simulink model "SingleTrack"  (Simulink 8.7)
settings: Solver=ode45  SolverMode=SingleTasking  StartTime=0.0  StopTime=inf  FixedStep=0.001  RelTol=1e-3
PreLoadFcn:
  | SingleTrack_params
undefined symbols (not defined in the file or in its folder): Car_Bdy1_mass, Car_Steering_i, Car_Whl_Radius, Car_WhlBaseF, Car_WhlBaseR, mEngineMax, PT_DL_iDiff, PT_GearBox_iForwardGears
libraries: CarMaker4SL x5
(part 2 of 4)

== system SingleTrack/CarMaker/Vehicle/IPG Vehicle/Brake/CreateBus Vhcl.Wheel.PT ==
  In : Inport
  BusCreator1 : BusCreator  Inputs=20
  Demux1 : Demux  Outputs=20
  Out : Outport
  wires:
  Demux1/20 -> BusCreator1/20  "Vhcl Trq_DriveSrc_trg d3"
  Demux1/19 -> BusCreator1/19  "Vhcl Trq_DriveSrc_trg d2"
  Demux1/18 -> BusCreator1/18  "Vhcl Trq_DriveSrc_trg d1"
  Demux1/17 -> BusCreator1/17  "Vhcl Trq_DriveSrc_trg d0"
  Demux1/16 -> BusCreator1/16  "Vhcl Wheel RR WhlBearing"
  Demux1/15 -> BusCreator1/15  "Vhcl Wheel RR Trq_T2W"
  Demux1/14 -> BusCreator1/14  "Vhcl Wheel RR Trq_BrakeReg_trg"
  Demux1/13 -> BusCreator1/13  "Vhcl Wheel RR Trq_Brake"
  Demux1/12 -> BusCreator1/12  "Vhcl Wheel RL WhlBearing"
  Demux1/11 -> BusCreator1/11  "Vhcl Wheel RL Trq_T2W"
  Demux1/10 -> BusCreator1/10  "Vhcl Wheel RL Trq_BrakeReg_trg"
  Demux1/9 -> BusCreator1/9  "Vhcl Wheel RL Trq_Brake"
  Demux1/8 -> BusCreator1/8  "Vhcl Wheel FR WhlBearing"
  Demux1/7 -> BusCreator1/7  "Vhcl Wheel FR Trq_T2W"
  Demux1/6 -> BusCreator1/6  "Vhcl Wheel FR Trq_BrakeReg_trg"
  Demux1/5 -> BusCreator1/5  "Vhcl Wheel FR Trq_Brake"
  Demux1/4 -> BusCreator1/4  "Vhcl Wheel FL WhlBearing"
  Demux1/3 -> BusCreator1/3  "Vhcl Wheel FL Trq_T2W"
  Demux1/2 -> BusCreator1/2  "Vhcl Wheel FL Trq_BrakeReg_trg"
  Demux1/1 -> BusCreator1/1  "Vhcl Wheel FL Trq_Brake"
  BusCreator1/1 -> Out/1
  In/1 -> Demux1/1

== system SingleTrack/CarMaker/Vehicle/IPG Vehicle/CarAndTrailer/CarAndTrailerUpd ==
  Sync_In : Inport
  Vhcl.Steering : Inport  Port=2
  Vhcl.Motion : Inport  Port=3
  Vhcl.PoI : Inport  Port=4
  Vhcl.Wheel.FL : Inport  Port=5
  Vhcl.Wheel.FR : Inport  Port=6
  Vhcl.Wheel.RL : Inport  Port=7
  Vhcl.Wheel.RR : Inport  Port=8
  Car.Hitch.FrcTrq : Inport  Port=9
  Vhcl.Fr1A : Inport  Port=10
  CarAndTrailerUpd : S-Function  FunctionName=CM_Sfun  Parameters='CarAndTrUpd'  SFunctionDeploymentMode=off  EnableBusSupport=off
  CreateBus Brake.IF.In : Subsystem
  Sync_Out : Outport
  Brake.IF.In : Outport  Port=2
  wires:
  Vhcl.Fr1A/1 -> CarAndTrailerUpd/10  "user vehicle only"
  Vhcl.Steering/1 -> CarAndTrailerUpd/2
  Vhcl.Motion/1 -> CarAndTrailerUpd/3
  Vhcl.PoI/1 -> CarAndTrailerUpd/4
  Vhcl.Wheel.FL/1 -> CarAndTrailerUpd/5
  Vhcl.Wheel.FR/1 -> CarAndTrailerUpd/6
  Car.Hitch.FrcTrq/1 -> CarAndTrailerUpd/9
  Vhcl.Wheel.RR/1 -> CarAndTrailerUpd/8
  Vhcl.Wheel.RL/1 -> CarAndTrailerUpd/7
  CarAndTrailerUpd/2 -> CreateBus Brake.IF.In/1(In)
  CreateBus Brake.IF.In/1(Out) -> Brake.IF.In/1
  CarAndTrailerUpd/1 -> Sync_Out/1
  Sync_In/1 -> CarAndTrailerUpd/1

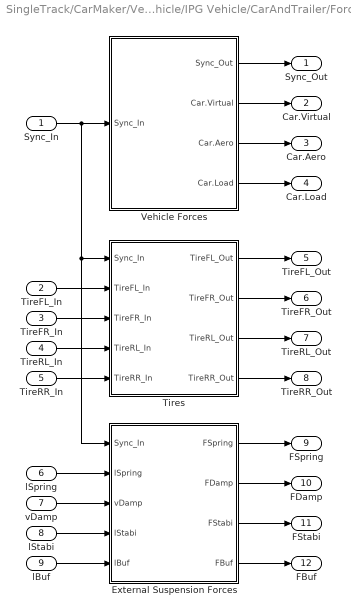
== system SingleTrack/CarMaker/Vehicle/IPG Vehicle/CarAndTrailer/Forces ==
  Sync_In : Inport
  TireFL_In : Inport  Port=2
  TireFR_In : Inport  Port=3
  TireRL_In : Inport  Port=4
  TireRR_In : Inport  Port=5
  lSpring : Inport  Port=6
  vDamp : Inport  Port=7
  lStabi : Inport  Port=8
  lBuf : Inport  Port=9
  External Suspension Forces : Subsystem
  Tires : Subsystem
  Vehicle Forces : Subsystem
  Sync_Out : Outport
  Car.Virtual : Outport  Port=2
  Car.Aero : Outport  Port=3
  Car.Load : Outport  Port=4
  TireFL_Out : Outport  Port=5
  TireFR_Out : Outport  Port=6
  TireRL_Out : Outport  Port=7
  TireRR_Out : Outport  Port=8
  FSpring : Outport  Port=9
  FDamp : Outport  Port=10
  FStabi : Outport  Port=11
  FBuf : Outport  Port=12
  wires:
  lBuf/1 -> External Suspension Forces/5(lBuf)
  lStabi/1 -> External Suspension Forces/4(lStabi)
  vDamp/1 -> External Suspension Forces/3(vDamp)
  Tires/4(TireRR_Out) -> TireRR_Out/1
  Tires/3(TireRL_Out) -> TireRL_Out/1
  Tires/2(TireFR_Out) -> TireFR_Out/1
  Tires/1(TireFL_Out) -> TireFL_Out/1
  TireRR_In/1 -> Tires/5(TireRR_In)
  TireRL_In/1 -> Tires/4(TireRL_In)
  TireFR_In/1 -> Tires/3(TireFR_In)
  TireFL_In/1 -> Tires/2(TireFL_In)
  External Suspension Forces/4(FBuf) -> FBuf/1
  Sync_In/1 -> External Suspension Forces/1(Sync_In), Tires/1(Sync_In), Vehicle Forces/1(Sync_In)
  Vehicle Forces/1(Sync_Out) -> Sync_Out/1
  Vehicle Forces/2(Car.Virtual) -> Car.Virtual/1
  Vehicle Forces/3(Car.Aero) -> Car.Aero/1
  Vehicle Forces/4(Car.Load) -> Car.Load/1
  lSpring/1 -> External Suspension Forces/2(lSpring)
  External Suspension Forces/2(FDamp) -> FDamp/1
  External Suspension Forces/3(FStabi) -> FStabi/1
  External Suspension Forces/1(FSpring) -> FSpring/1

== system SingleTrack/CarMaker/Vehicle/IPG Vehicle/CarAndTrailer/Kinematics ==
  Sync_In : Inport
  Steer.IF : Inport  Port=2
  Kinematics : S-Function  FunctionName=CM_Sfun  Parameters='Kinematics'  SFunctionDeploymentMode=off  EnableBusSupport=off
  Sync_Out : Outport
  TireFL_In : Outport  Port=2
  TireFR_In : Outport  Port=3
  TireRL_In : Outport  Port=4
  TireRR_In : Outport  Port=5
  lSpring : Outport  Port=6
  vDamp : Outport  Port=7
  lStabi : Outport  Port=8
  lBuf : Outport  Port=9
  wires:
  Kinematics/9 -> lBuf/1
  Kinematics/8 -> lStabi/1
  Kinematics/2 -> TireFL_In/1
  Kinematics/3 -> TireFR_In/1
  Kinematics/4 -> TireRL_In/1
  Kinematics/5 -> TireRR_In/1
  Kinematics/6 -> lSpring/1
  Kinematics/7 -> vDamp/1
  Sync_In/1 -> Kinematics/1
  Kinematics/1 -> Sync_Out/1
  Steer.IF/1 -> Kinematics/2

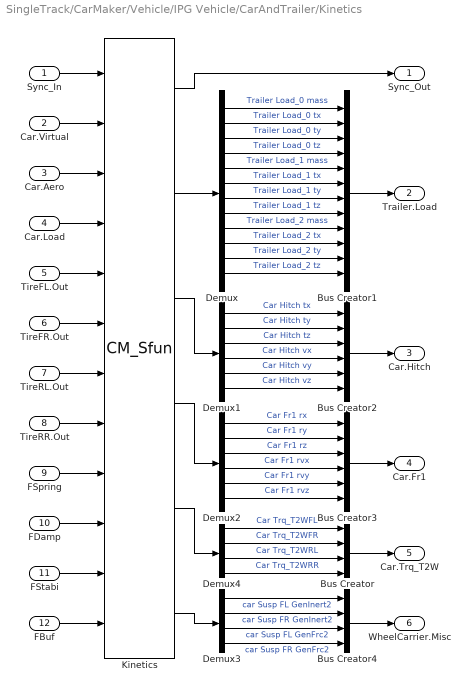
== system SingleTrack/CarMaker/Vehicle/IPG Vehicle/CarAndTrailer/Kinetics ==
  Sync_In : Inport
  Car.Virtual : Inport  Port=2
  Car.Aero : Inport  Port=3
  Car.Load : Inport  Port=4
  TireFL.Out : Inport  Port=5
  TireFR.Out : Inport  Port=6
  TireRL.Out : Inport  Port=7
  TireRR.Out : Inport  Port=8
  FSpring : Inport  Port=9
  FDamp : Inport  Port=10
  FStabi : Inport  Port=11
  FBuf : Inport  Port=12
  Bus Creator : BusCreator  Inputs=4
  Bus Creator1 : BusCreator  Inputs=12
  Bus Creator2 : BusCreator  Inputs=6
  Bus Creator3 : BusCreator  Inputs=6
  Bus Creator4 : BusCreator  Inputs=4
  Demux : Demux  Outputs=12
  Demux1 : Demux  Outputs=6
  Demux2 : Demux  Outputs=6
  Demux3 : Demux
  Demux4 : Demux
  Kinetics : S-Function  FunctionName=CM_Sfun  Parameters='Kinetics'  SFunctionDeploymentMode=off  EnableBusSupport=off
  Sync_Out : Outport
  Trailer.Load : Outport  Port=2
  Car.Hitch : Outport  Port=3
  Car.Fr1 : Outport  Port=4
  Car.Trq_T2W : Outport  Port=5
  WheelCarrier.Misc : Outport  Port=6
  wires:
  FBuf/1 -> Kinetics/12
  Sync_In/1 -> Kinetics/1
  Kinetics/1 -> Sync_Out/1
  Car.Aero/1 -> Kinetics/3
  Car.Virtual/1 -> Kinetics/2
  Bus Creator1/1 -> Trailer.Load/1
  Demux/1 -> Bus Creator1/1  "Trailer Load_0 mass"
  Demux/2 -> Bus Creator1/2  "Trailer Load_0 tx"
  Demux/3 -> Bus Creator1/3  "Trailer Load_0 ty"
  Demux/4 -> Bus Creator1/4  "Trailer Load_0 tz"
  Kinetics/2 -> Demux/1
  Demux/5 -> Bus Creator1/5  "Trailer Load_1 mass"
  Demux/6 -> Bus Creator1/6  "Trailer Load_1 tx"
  Demux/7 -> Bus Creator1/7  "Trailer Load_1 ty"
  Demux/8 -> Bus Creator1/8  "Trailer Load_1 tz"
  Demux/9 -> Bus Creator1/9  "Trailer Load_2 mass"
  Demux/10 -> Bus Creator1/10  "Trailer Load_2 tx"
  Demux/11 -> Bus Creator1/11  "Trailer Load_2 ty"
  Demux/12 -> Bus Creator1/12  "Trailer Load_2 tz"
  Demux1/1 -> Bus Creator2/1  "Car Hitch tx"
  Demux1/2 -> Bus Creator2/2  "Car Hitch ty"
  Demux1/3 -> Bus Creator2/3  "Car Hitch tz"
  Demux1/4 -> Bus Creator2/4  "Car Hitch vx"
  Demux1/5 -> Bus Creator2/5  "Car Hitch vy"
  Demux1/6 -> Bus Creator2/6  "Car Hitch vz"
  Kinetics/3 -> Demux1/1
  Bus Creator2/1 -> Car.Hitch/1
  Demux2/1 -> Bus Creator3/1  "Car Fr1 rx"
  Demux2/2 -> Bus Creator3/2  "Car Fr1 ry"
  Demux2/3 -> Bus Creator3/3  "Car Fr1 rz"
  Demux2/4 -> Bus Creator3/4  "Car Fr1 rvx"
  Demux2/5 -> Bus Creator3/5  "Car Fr1 rvy"
  Demux2/6 -> Bus Creator3/6  "Car Fr1 rvz"
  Bus Creator3/1 -> Car.Fr1/1
  Kinetics/4 -> Demux2/1
  Car.Load/1 -> Kinetics/4
  Demux3/1 -> Bus Creator4/1  "car Susp FL GenInert2"
  Demux3/2 -> Bus Creator4/2  "car Susp FR GenInert2"
  Demux3/3 -> Bus Creator4/3  "car Susp FL GenFrc2"
  Demux3/4 -> Bus Creator4/4  "car Susp FR GenFrc2"
  Bus Creator4/1 -> WheelCarrier.Misc/1
  Bus Creator/1 -> Car.Trq_T2W/1
  Demux4/4 -> Bus Creator/4  "Car Trq_T2WRR"
  Demux4/3 -> Bus Creator/3  "Car Trq_T2WRL"
  Demux4/2 -> Bus Creator/2  "Car Trq_T2WFR"
  Demux4/1 -> Bus Creator/1  "Car Trq_T2WFL"
  TireFL.Out/1 -> Kinetics/5
  TireFR.Out/1 -> Kinetics/6
  TireRL.Out/1 -> Kinetics/7
  TireRR.Out/1 -> Kinetics/8
  FSpring/1 -> Kinetics/9
  FDamp/1 -> Kinetics/10
  FStabi/1 -> Kinetics/11
  Kinetics/6 -> Demux3/1
  Kinetics/5 -> Demux4/1

== system SingleTrack/CarMaker/Vehicle/IPG Vehicle/CarAndTrailer/Steering ==
  note: When replacing the entire steering system,
      | be sure to disable the IPG steering model by using the steering
      | model 'Model Manager off' in the vehicle GUI.
  Sync_In : Inport
  VhclCtrl.Steering : Inport  Port=2
  Bus Creator1 : BusCreator  Inputs=16
  Bus Creator2 : BusCreator  Inputs=5
  Demux : Demux  Outputs=21
  Steering : S-Function  FunctionName=CM_Sfun  Parameters='Steering'  SFunctionDeploymentMode=off  EnableBusSupport=off
  Terminator : Terminator
  Sync_Out : Outport
  Steer.IF : Outport  Port=2
  wires:
  Demux/21 -> Bus Creator2/5  "Steering IF R Inert"
  Demux/20 -> Bus Creator2/4  "Steering IF R Frc"
  Demux/19 -> Bus Creator2/3  "Steering IF L Inert"
  Demux/18 -> Bus Creator2/2  "Steering IF L Frc"
  Demux/17 -> Bus Creator2/1  "Steering IF SteerByTrq"
  Demux/16 -> Bus Creator1/16  "Steering IF R iSteer2q"
  Demux/15 -> Bus Creator1/15  "Steering IF R qpp"
  Demux/14 -> Bus Creator1/14  "Steering IF R qp"
  Demux/13 -> Bus Creator1/13  "Steering IF R q"
  Demux/12 -> Bus Creator1/12  "Steering IF L iSteer2q"
  Demux/11 -> Bus Creator1/11  "Steering IF L qpp"
  Demux/10 -> Bus Creator1/10  "Steering IF L qp"
  Demux/9 -> Bus Creator1/9  "Steering IF L q"
  Demux/8 -> Bus Creator1/8  "Steering IF AssistTrqPin"
  Demux/7 -> Bus Creator1/7  "Steering IF AssistTrqCol"
  Demux/6 -> Bus Creator1/6  "Steering IF AssistFrc"
  Demux/5 -> Bus Creator1/5  "Steering IF TrqStatic"
  Demux/4 -> Bus Creator1/4  "Steering IF Trq"
  Demux/3 -> Bus Creator1/3  "Steering IF AngAcc"
  Demux/2 -> Bus Creator1/2  "Steering IF AngVel"
  Demux/1 -> Bus Creator1/1  "Steering IF Ang"
  Bus Creator1/1 -> Steer.IF/1
  Steering/2 -> Demux/1
  Bus Creator2/1 -> Terminator/1  "Steer IF (in)"
  VhclCtrl.Steering/1 -> Steering/2
  Steering/1 -> Sync_Out/1
  Sync_In/1 -> Steering/1

== system SingleTrack/CarMaker/Vehicle/IPG Vehicle/CarAndTrailer/Trailer ==
  Sync_In : Inport
  Trailer.Load : Inport  Port=2
  Car.Hitch : Inport  Port=3
  Car.Fr1 : Inport  Port=4
  Car.Trq_T2W : Inport  Port=5
  WheelCarrier.Misc : Inport  Port=6
  CreateBus Car.Hitch.FrcTrq : Subsystem
  CreateBus Vhcl.Motion : Subsystem
  CreateBus Vhcl.PoI : Subsystem
  CreateBus Vhcl.Steering : Subsystem
  CreateBus Vhcl.Wheel.FL : Subsystem
  CreateBus Vhcl.Wheel.FR : Subsystem
  CreateBus Vhcl.Wheel.RL : Subsystem
  CreateBus Vhcl.Wheel.RR : Subsystem
  Trailer : S-Function  FunctionName=CM_Sfun  Parameters='Trailer'  SFunctionDeploymentMode=off  EnableBusSupport=off
  Sync_Out : Outport
  Vhcl.Steering : Outport  Port=2
  Vhcl.Motion : Outport  Port=3
  Vhcl.PoI : Outport  Port=4
  Vhcl.Wheel.FL : Outport  Port=5
  Vhcl.Wheel.FR : Outport  Port=6
  Vhcl.Wheel.RL : Outport  Port=7
  Vhcl.Wheel.RR : Outport  Port=8
  Car.Hitch.FrcTrq : Outport  Port=9
  wires:
  Trailer/2 -> CreateBus Vhcl.Steering/1(In1)
  CreateBus Vhcl.Steering/1(Out1) -> Vhcl.Steering/1  "Vhcl.Steering"
  Trailer/3 -> CreateBus Vhcl.Motion/1(In1)
  Trailer/4 -> CreateBus Vhcl.PoI/1(In1)
  Trailer/5 -> CreateBus Vhcl.Wheel.FL/1(In1)
  Trailer/6 -> CreateBus Vhcl.Wheel.FR/1(In1)
  Trailer/7 -> CreateBus Vhcl.Wheel.RL/1(In1)
  Trailer/9 -> CreateBus Car.Hitch.FrcTrq/1(In1)
  Trailer/8 -> CreateBus Vhcl.Wheel.RR/1(In1)
  CreateBus Vhcl.Wheel.RR/1(Out1) -> Vhcl.Wheel.RR/1  "Vhcl.Wheel.RR"
  CreateBus Vhcl.Wheel.RL/1(Out1) -> Vhcl.Wheel.RL/1  "Vhcl.Wheel.RL"
  CreateBus Vhcl.Wheel.FR/1(Out1) -> Vhcl.Wheel.FR/1  "Vhcl.Wheel.FR"
  CreateBus Vhcl.Wheel.FL/1(Out1) -> Vhcl.Wheel.FL/1  "Vhcl.Wheel.FL"
  CreateBus Vhcl.PoI/1(Out1) -> Vhcl.PoI/1  "Vhcl.PoI"
  CreateBus Vhcl.Motion/1(Out1) -> Vhcl.Motion/1  "Vhcl.Motion"
  Car.Trq_T2W/1 -> Trailer/5
  WheelCarrier.Misc/1 -> Trailer/6
  CreateBus Car.Hitch.FrcTrq/1(Out1) -> Car.Hitch.FrcTrq/1  "Car.Hitch.FrcTrq"
  Car.Fr1/1 -> Trailer/4
  Car.Hitch/1 -> Trailer/3
  Trailer.Load/1 -> Trailer/2
  Trailer/1 -> Sync_Out/1
  Sync_In/1 -> Trailer/1

== system SingleTrack/CarMaker/Vehicle/User Vehicle (CM4SL)/Brake/CreateBus Vhcl.Wheel.PT ==
  In : Inport
  BusCreator1 : BusCreator  Inputs=20
  Demux1 : Demux  Outputs=20
  Out : Outport
  wires:
  Demux1/20 -> BusCreator1/20  "Vhcl Trq_DriveSrc_trg d3"
  Demux1/19 -> BusCreator1/19  "Vhcl Trq_DriveSrc_trg d2"
  Demux1/18 -> BusCreator1/18  "Vhcl Trq_DriveSrc_trg d1"
  Demux1/17 -> BusCreator1/17  "Vhcl Trq_DriveSrc_trg d0"
  Demux1/16 -> BusCreator1/16  "Vhcl Wheel RR WhlBearing"
  Demux1/15 -> BusCreator1/15  "Vhcl Wheel RR Trq_T2W"
  Demux1/14 -> BusCreator1/14  "Vhcl Wheel RR Trq_BrakeReg_trg"
  Demux1/13 -> BusCreator1/13  "Vhcl Wheel RR Trq_Brake"
  Demux1/12 -> BusCreator1/12  "Vhcl Wheel RL WhlBearing"
  Demux1/11 -> BusCreator1/11  "Vhcl Wheel RL Trq_T2W"
  Demux1/10 -> BusCreator1/10  "Vhcl Wheel RL Trq_BrakeReg_trg"
  Demux1/9 -> BusCreator1/9  "Vhcl Wheel RL Trq_Brake"
  Demux1/8 -> BusCreator1/8  "Vhcl Wheel FR WhlBearing"
  Demux1/7 -> BusCreator1/7  "Vhcl Wheel FR Trq_T2W"
  Demux1/6 -> BusCreator1/6  "Vhcl Wheel FR Trq_BrakeReg_trg"
  Demux1/5 -> BusCreator1/5  "Vhcl Wheel FR Trq_Brake"
  Demux1/4 -> BusCreator1/4  "Vhcl Wheel FL WhlBearing"
  Demux1/3 -> BusCreator1/3  "Vhcl Wheel FL Trq_T2W"
  Demux1/2 -> BusCreator1/2  "Vhcl Wheel FL Trq_BrakeReg_trg"
  Demux1/1 -> BusCreator1/1  "Vhcl Wheel FL Trq_Brake"
  BusCreator1/1 -> Out/1
  In/1 -> Demux1/1

== system SingleTrack/CarMaker/Vehicle/User Vehicle (CM4SL)/CarAndTrailer/CarAndTrailerUpd ==
  Sync_In : Inport
  Vhcl.Steering : Inport  Port=2
  Vhcl.Motion : Inport  Port=3
  Vhcl.PoI : Inport  Port=4
  Vhcl.Wheel.FL : Inport  Port=5
  Vhcl.Wheel.FR : Inport  Port=6
  Vhcl.Wheel.RL : Inport  Port=7
  Vhcl.Wheel.RR : Inport  Port=8
  Car.Hitch.FrcTrq : Inport  Port=9
  Vhcl.Fr1A : Inport  Port=10
  CarAndTrailerUpd : S-Function  FunctionName=CM_Sfun  Parameters='CarAndTrUpd'  SFunctionDeploymentMode=off  EnableBusSupport=off
  CreateBus Brake.IF.In : Subsystem
  Sync_Out : Outport
  Brake.IF.In : Outport  Port=2
  wires:
  Vhcl.Fr1A/1 -> CarAndTrailerUpd/10  "user vehicle only"
  Vhcl.Steering/1 -> CarAndTrailerUpd/2
  Vhcl.Motion/1 -> CarAndTrailerUpd/3
  Vhcl.PoI/1 -> CarAndTrailerUpd/4
  Vhcl.Wheel.FL/1 -> CarAndTrailerUpd/5
  Vhcl.Wheel.FR/1 -> CarAndTrailerUpd/6
  Car.Hitch.FrcTrq/1 -> CarAndTrailerUpd/9
  Vhcl.Wheel.RR/1 -> CarAndTrailerUpd/8
  Vhcl.Wheel.RL/1 -> CarAndTrailerUpd/7
  CarAndTrailerUpd/2 -> CreateBus Brake.IF.In/1(In)
  CreateBus Brake.IF.In/1(Out) -> Brake.IF.In/1
  CarAndTrailerUpd/1 -> Sync_Out/1
  Sync_In/1 -> CarAndTrailerUpd/1

== system SingleTrack/CarMaker/Vehicle/User Vehicle (CM4SL)/CarAndTrailer/CreateBus Car.Hitch.FrcTrq ==
  Bus Creator : BusCreator  Inputs=6
  Constant{1..2,7..10} (6 alike) : Constant  Value=0
  Demux7 : Demux  Outputs=6
  Mux1 : Mux  Inputs=6
  Car.Hitch.FrcTrq : Outport
  wires:
  Constant1/1 -> Mux1/6
  Constant2/1 -> Mux1/5
  Constant7/1 -> Mux1/1
  Constant10/1 -> Mux1/4
  Constant9/1 -> Mux1/3
  Constant8/1 -> Mux1/2
  Mux1/1 -> Demux7/1
  Bus Creator/1 -> Car.Hitch.FrcTrq/1
  Demux7/6 -> Bus Creator/6  "Car Hitch Trq2Car z"
  Demux7/5 -> Bus Creator/5  "Car Hitch Trq2Car y"
  Demux7/4 -> Bus Creator/4  "Car Hitch Trq2Car x"
  Demux7/3 -> Bus Creator/3  "Car Hitch Frc2Car z"
  Demux7/2 -> Bus Creator/2  "Car Hitch Frc2Car y"
  Demux7/1 -> Bus Creator/1  "Car Hitch Frc2Car x"

== system SingleTrack/CarMaker/Vehicle/User Vehicle (CM4SL)/CarAndTrailer/CreateBus Vhcl.Fr1 ==
  Vhcl.Fr1_In : Inport
  BdyFrame2Vhcl.Fr1A : Subsystem
  Ground : Ground
  Ground1 : Ground
  Tr2Fr0 : Subsystem
  a_0 : Subsystem
  t_0 : Subsystem
  v_0 : Subsystem
  Vhcl.Fr1A : Outport
  wires:
  Ground/1 -> BdyFrame2Vhcl.Fr1A/5(alpha_0)
  Ground1/1 -> BdyFrame2Vhcl.Fr1A/4(omega_0)
  a_0/1(a_0) -> BdyFrame2Vhcl.Fr1A/3(a_0)
  v_0/1(v_0) -> BdyFrame2Vhcl.Fr1A/2(v_0)
  t_0/1(t_0) -> BdyFrame2Vhcl.Fr1A/1(t_0)
  Tr2Fr0/1(Tr2Fr0) -> BdyFrame2Vhcl.Fr1A/6(Tr2Fr0), a_0/2(Tr2Fr0), v_0/2(Tr2Fr0)
  Vhcl.Fr1_In/1 -> Tr2Fr0/1(Car), t_0/1(Car), v_0/1(Car), a_0/1(Car)
  BdyFrame2Vhcl.Fr1A/1(Vhcl.Fr1) -> Vhcl.Fr1A/1

== system SingleTrack/CarMaker/Vehicle/User Vehicle (CM4SL)/CarAndTrailer/CreateBus Vhcl.Motion ==
  Vhcl_Motion_In : Inport
  Bus Selector1 : BusSelector  OutputSignals=Car_vx_1,Car_Dist,Car_sRoad,Road_Fr1_rx,Road_Fr1_ry,Car_Yaw,Car_Yawp,Car_Yawpp
  BusCreator : BusCreator  Inputs=15
  Constant{1,5,8,11..14} (7 alike) : Constant  Value=0
  Demux : Demux  Outputs=15
  Mux3 : Mux  Inputs=15
  Vhcl .Motion : Outport
  wires:
  Bus Selector1/1 -> Mux3/1  "<Car_vx_1>"
  Bus Selector1/2 -> Mux3/2  "<Car_Dist>"
  Constant5/1 -> Mux3/4
  Constant8/1 -> Mux3/5
  Constant11/1 -> Mux3/6
  Constant12/1 -> Mux3/8
  Constant13/1 -> Mux3/9
  Constant14/1 -> Mux3/11
  Constant1/1 -> Mux3/12
  Bus Selector1/7 -> Mux3/14  "<Car_Yawp>"
  Bus Selector1/8 -> Mux3/15  "<Car_Yawpp>"
  Bus Selector1/4 -> Mux3/7  "<Road_Fr1_rx>"
  Bus Selector1/5 -> Mux3/10  "<Road_Fr1_ry>"
  Bus Selector1/3 -> Mux3/3  "<Car_sRoad>"
  BusCreator/1 -> Vhcl .Motion/1
  Mux3/1 -> Demux/1
  Vhcl_Motion_In/1 -> Bus Selector1/1
  Demux/1 -> BusCreator/1  "Vhcl v"
  Demux/2 -> BusCreator/2  "Vhcl Distance"
  Demux/3 -> BusCreator/3  "Vhcl sRoad"
  Demux/4 -> BusCreator/4  "Vhcl Hitch_Pos x"
  Demux/5 -> BusCreator/5  "Vhcl Hitch_Pos y"
  Demux/6 -> BusCreator/6  "Vhcl Hitch_Pos z"
  Demux/7 -> BusCreator/7  "Vhcl Roll"
  Demux/8 -> BusCreator/8  "Vhcl RollVel"
  Demux/9 -> BusCreator/9  "Vhcl RollAcc"
  Demux/10 -> BusCreator/10  "Vhcl Pitch"
  Demux/11 -> BusCreator/11  "Vhcl PitchVel"
  Demux/12 -> BusCreator/12  "Vhcl PitchAcc"
  Demux/13 -> BusCreator/13  "Vhcl Yaw"
  Demux/14 -> BusCreator/14  "Vhcl YawVel"
  Demux/15 -> BusCreator/15  "Vhcl YawAcc"
  Bus Selector1/6 -> Mux3/13  "<Car_Yaw>"

== system SingleTrack/CarMaker/Vehicle/User Vehicle (CM4SL)/CarAndTrailer/CreateBus Vhcl.PoI ==
  Vhcl_POI_In : Inport
  Bus Creator : BusCreator  Inputs=18
  Bus Selector : BusSelector  OutputSignals=Car_x,Car_y,Road_Fr1_z,Car_vx,Car_vy,Car_ax,Car_ay,Car_vx_1,Car_ax_1,Car_ay_1
  Constant{11..13,15..19} (8 alike) : Constant  Value=0
  Demux3 : Demux  Outputs=18
  Mux1 : Mux  Inputs=18
  Vhcl.PoI : Outport
  wires:
  Bus Selector/8 -> Mux1/10  "<Car_vx_1>"
  Bus Selector/7 -> Mux1/8  "<Car_ay>"
  Constant19/1 -> Mux1/15
  Bus Selector/10 -> Mux1/14  "<Car_ay_1>"
  Bus Selector/9 -> Mux1/13  "<Car_ax_1>"
  Constant18/1 -> Mux1/12
  Constant17/1 -> Mux1/11
  Constant16/1 -> Mux1/9
  Bus Selector/6 -> Mux1/7  "<Car_ax>"
  Constant15/1 -> Mux1/6
  Bus Selector/5 -> Mux1/5  "<Car_vy>"
  Bus Selector/4 -> Mux1/4  "<Car_vx>"
  Bus Selector/3 -> Mux1/3  "<Road_Fr1_z>"
  Bus Selector/2 -> Mux1/2  "<Car_y>"
  Bus Selector/1 -> Mux1/1  "<Car_x>"
  Constant11/1 -> Mux1/18
  Constant13/1 -> Mux1/17
  Constant12/1 -> Mux1/16
  Vhcl_POI_In/1 -> Bus Selector/1
  Mux1/1 -> Demux3/1
  Demux3/18 -> Bus Creator/18  "Vhcl PoI_GCS Elev"
  Demux3/17 -> Bus Creator/17  "Vhcl PoI_GCS Lat"
  Demux3/16 -> Bus Creator/16  "Vhcl PoI_GCS Long"
  Demux3/15 -> Bus Creator/15  "Vhcl PoI_Acc_1 z"
  Demux3/14 -> Bus Creator/14  "Vhcl PoI_Acc_1 y"
  Demux3/13 -> Bus Creator/13  "Vhcl PoI_Acc_1 x"
  Demux3/12 -> Bus Creator/12  "Vhcl PoI_Vel_1 z"
  Demux3/11 -> Bus Creator/11  "Vhcl PoI_Vel_1 y"
  Demux3/10 -> Bus Creator/10  "Vhcl PoI_Vel_1 x"
  Demux3/9 -> Bus Creator/9  "Vhcl PoI_Acc z"
  Demux3/8 -> Bus Creator/8  "Vhcl PoI_Acc y"
  Demux3/7 -> Bus Creator/7  "Vhcl PoI_Acc x"
  Demux3/6 -> Bus Creator/6  "Vhcl PoI_Vel z"
  Demux3/5 -> Bus Creator/5  "Vhcl PoI_Vel y"
  Demux3/4 -> Bus Creator/4  "Vhcl PoI_Vel x"
  Demux3/3 -> Bus Creator/3  "Vhcl PoI_Pos z"
  Demux3/2 -> Bus Creator/2  "Vhcl PoI_Pos y"
  Bus Creator/1 -> Vhcl.PoI/1
  Demux3/1 -> Bus Creator/1  "Vhcl PoI_Pos x"

== system SingleTrack/CarMaker/Vehicle/User Vehicle (CM4SL)/CarAndTrailer/CreateBus Vhcl.Steering ==
  Vhcl_Steering_In : Inport
  Bus Creator : BusCreator  Inputs=4
  Bus Selector : BusSelector  OutputSignals=VhclCtrl Steering Ang,VhclCtrl Steering AngVel,VhclCtrl Steering AngAcc,VhclCtrl Steering Trq
  Demux : Demux
  Mux1 : Mux
  Vhcl.Steering : Outport
  wires:
  Mux1/1 -> Demux/1
  Bus Selector/4 -> Mux1/4  "<VhclCtrl Steering Trq>"
  Bus Selector/3 -> Mux1/3  "<VhclCtrl Steering AngAcc>"
  Bus Selector/2 -> Mux1/2  "<VhclCtrl Steering AngVel>"
  Bus Selector/1 -> Mux1/1  "<VhclCtrl Steering Ang>"
  Vhcl_Steering_In/1 -> Bus Selector/1
  Bus Creator/1 -> Vhcl.Steering/1
  Demux/1 -> Bus Creator/1  "Vhcl Steering Ang"
  Demux/3 -> Bus Creator/3  "Vhcl Steering AngAcc"
  Demux/2 -> Bus Creator/2  "Vhcl Steering AngVel"
  Demux/4 -> Bus Creator/4  "Vhcl Steering Trq"

== system SingleTrack/CarMaker/Vehicle/User Vehicle (CM4SL)/CarAndTrailer/CreateBus Vhcl.Wheel.FL ==
  Vhcl.Wheel.FL_In : Inport
  Bus Creator : BusCreator  Inputs=14
  Bus Selector : BusSelector  OutputSignals=Car_Whl_F_rz,Car_Whl_Fz,Car_Whl_F_SideSlip
  Constant{1..6,8..12} (11 alike) : Constant  Value=0
  Demux3 : Demux  Outputs=14
  Mux1 : Mux  Inputs=14
  Vhcl.Wheel.FL : Outport
  wires:
  Bus Selector/2 -> Mux1/9  "<Car_Whl_Fz>"
  Constant11/1 -> Mux1/14
  Constant12/1 -> Mux1/13
  Constant10/1 -> Mux1/11
  Constant9/1 -> Mux1/10
  Bus Selector/3 -> Mux1/12  "<Car_Whl_F_SideSlip>"
  Constant8/1 -> Mux1/8
  Constant6/1 -> Mux1/7
  Constant5/1 -> Mux1/5
  Constant4/1 -> Mux1/4
  Constant3/1 -> Mux1/3
  Constant2/1 -> Mux1/2
  Constant1/1 -> Mux1/1
  Bus Selector/1 -> Mux1/6  "<Car_Whl_F_rz>"
  Vhcl.Wheel.FL_In/1 -> Bus Selector/1
  Demux3/14 -> Bus Creator/14  "Vhcl Wheel FL Trq_WhlBearing"
  Demux3/13 -> Bus Creator/13  "Vhcl Wheel FL Trq_T2W"
  Demux3/12 -> Bus Creator/12  "Vhcl Wheel FL SideSlip"
  Demux3/11 -> Bus Creator/11  "Vhcl Wheel FL LongSlip"
  Demux3/10 -> Bus Creator/10  "Vhcl Wheel FL vBelt"
  Demux3/9 -> Bus Creator/9  "Vhcl Wheel FL Fz"
  Demux3/8 -> Bus Creator/8  "Vhcl Wheel FL Fy"
  Demux3/7 -> Bus Creator/7  "Vhcl Wheel FL Fx"
  Demux3/6 -> Bus Creator/6  "Vhcl Wheel FL r_zxy z"
  Demux3/5 -> Bus Creator/5  "Vhcl Wheel FL r_zxy y"
  Demux3/4 -> Bus Creator/4  "Vhcl Wheel FL r_zxy x"
  Demux3/3 -> Bus Creator/3  "Vhcl Wheel FL t z"
  Demux3/2 -> Bus Creator/2  "Vhcl Wheel FL t y"
  Mux1/1 -> Demux3/1
  Bus Creator/1 -> Vhcl.Wheel.FL/1
  Demux3/1 -> Bus Creator/1  "Vhcl Wheel FL t x"

== system SingleTrack/CarMaker/Vehicle/User Vehicle (CM4SL)/CarAndTrailer/CreateBus Vhcl.Wheel.FR ==
  Vhcl.Wheel.FR_In : Inport
  Bus Creator : BusCreator  Inputs=14
  Bus Selector : BusSelector  OutputSignals=Car_Whl_F_rz,Car_Whl_Fz,Car_Whl_F_SideSlip
  Constant{1..7,9..12} (11 alike) : Constant  Value=0
  Demux3 : Demux  Outputs=14
  Mux1 : Mux  Inputs=14
  Vhcl.Wheel.FR : Outport
  wires:
  Constant11/1 -> Mux1/14
  Constant12/1 -> Mux1/13
  Constant10/1 -> Mux1/11
  Constant9/1 -> Mux1/10
  Bus Selector/3 -> Mux1/12  "<Car_Whl_F_SideSlip>"
  Bus Selector/2 -> Mux1/9  "<Car_Whl_Fz>"
  Constant7/1 -> Mux1/8
  Constant6/1 -> Mux1/7
  Constant5/1 -> Mux1/5
  Constant4/1 -> Mux1/4
  Constant3/1 -> Mux1/3
  Constant2/1 -> Mux1/2
  Constant1/1 -> Mux1/1
  Bus Selector/1 -> Mux1/6  "<Car_Whl_F_rz>"
  Vhcl.Wheel.FR_In/1 -> Bus Selector/1
  Mux1/1 -> Demux3/1
  Demux3/14 -> Bus Creator/14  "Vhcl Wheel FR Trq_WhlBearing"
  Demux3/13 -> Bus Creator/13  "Vhcl Wheel FR Trq_T2W"
  Demux3/12 -> Bus Creator/12  "Vhcl Wheel FR SideSlip"
  Demux3/11 -> Bus Creator/11  "Vhcl Wheel FR LongSlip"
  Demux3/10 -> Bus Creator/10  "Vhcl Wheel FR vBelt"
  Demux3/9 -> Bus Creator/9  "Vhcl Wheel FR Fz"
  Demux3/8 -> Bus Creator/8  "Vhcl Wheel FR Fy"
  Demux3/7 -> Bus Creator/7  "Vhcl Wheel FR Fx"
  Demux3/6 -> Bus Creator/6  "Vhcl Wheel FR r_zxy z"
  Demux3/5 -> Bus Creator/5  "Vhcl Wheel FR r_zxy y"
  Demux3/4 -> Bus Creator/4  "Vhcl Wheel FR r_zxy x"
  Demux3/3 -> Bus Creator/3  "Vhcl Wheel FR t z"
  Demux3/2 -> Bus Creator/2  "Vhcl Wheel FR t y"
  Bus Creator/1 -> Vhcl.Wheel.FR/1
  Demux3/1 -> Bus Creator/1  "Vhcl Wheel FR t x"

== system SingleTrack/CarMaker/Vehicle/User Vehicle (CM4SL)/CarAndTrailer/CreateBus Vhcl.Wheel.RL ==
  Vhcl.Wheel.RL_In : Inport
  Bus Creator : BusCreator  Inputs=14
  Bus Selector : BusSelector  OutputSignals=Car_Whl_Fz,Car_Whl_R_SideSlip
  Constant{1..7,9..13} (12 alike) : Constant  Value=0
  Demux3 : Demux  Outputs=14
  Mux1 : Mux  Inputs=14
  Vhcl.Wheel.RL : Outport
  wires:
  Bus Selector/2 -> Mux1/12  "<Car_Whl_R_SideSlip>"
  Constant13/1 -> Mux1/6
  Constant11/1 -> Mux1/14
  Constant12/1 -> Mux1/13
  Constant10/1 -> Mux1/11
  Constant9/1 -> Mux1/10
  Bus Selector/1 -> Mux1/9  "<Car_Whl_Fz>"
  Constant7/1 -> Mux1/8
  Constant6/1 -> Mux1/7
  Constant5/1 -> Mux1/5
  Constant4/1 -> Mux1/4
  Constant3/1 -> Mux1/3
  Constant2/1 -> Mux1/2
  Constant1/1 -> Mux1/1
  Vhcl.Wheel.RL_In/1 -> Bus Selector/1
  Mux1/1 -> Demux3/1
  Demux3/14 -> Bus Creator/14  "Vhcl Wheel RL Trq_WhlBearing"
  Demux3/13 -> Bus Creator/13  "Vhcl Wheel RL Trq_T2W"
  Demux3/12 -> Bus Creator/12  "Vhcl Wheel RL SideSlip"
  Demux3/11 -> Bus Creator/11  "Vhcl Wheel RL LongSlip"
  Demux3/10 -> Bus Creator/10  "Vhcl Wheel RL vBelt"
  Demux3/9 -> Bus Creator/9  "Vhcl Wheel RL Fz"
  Demux3/8 -> Bus Creator/8  "Vhcl Wheel RL Fy"
  Demux3/7 -> Bus Creator/7  "Vhcl Wheel RL Fx"
  Demux3/6 -> Bus Creator/6  "Vhcl Wheel RL r_zxy z"
  Demux3/5 -> Bus Creator/5  "Vhcl Wheel RL r_zxy y"
  Demux3/4 -> Bus Creator/4  "Vhcl Wheel RL r_zxy x"
  Demux3/3 -> Bus Creator/3  "Vhcl Wheel RL t z"
  Demux3/2 -> Bus Creator/2  "Vhcl Wheel RL t y"
  Bus Creator/1 -> Vhcl.Wheel.RL/1
  Demux3/1 -> Bus Creator/1  "Vhcl Wheel RL t x"

== system SingleTrack/CarMaker/Vehicle/User Vehicle (CM4SL)/CarAndTrailer/CreateBus Vhcl.Wheel.RR ==
  Vhcl.Wheel.RR_In : Inport
  Bus Selector : BusSelector  OutputSignals=Car_Whl_Fz,Car_Whl_R_SideSlip
  Constant{1..7,9..13} (12 alike) : Constant  Value=0
  Demux3 : Demux  Outputs=14
  Mux : Mux  Inputs=14
  Mux1 : Mux  Inputs=14
  Vhcl.Wheel.RR : Outport
  wires:
  Bus Selector/2 -> Mux1/12  "<Car_Whl_R_SideSlip>"
  Constant13/1 -> Mux1/6
  Constant11/1 -> Mux1/14
  Constant12/1 -> Mux1/13
  Constant10/1 -> Mux1/11
  Constant9/1 -> Mux1/10
  Bus Selector/1 -> Mux1/9  "<Car_Whl_Fz>"
  Constant7/1 -> Mux1/8
  Constant6/1 -> Mux1/7
  Constant5/1 -> Mux1/5
  Constant4/1 -> Mux1/4
  Constant3/1 -> Mux1/3
  Constant2/1 -> Mux1/2
  Constant1/1 -> Mux1/1
  Vhcl.Wheel.RR_In/1 -> Bus Selector/1
  Mux1/1 -> Demux3/1
  Demux3/14 -> Mux/14  "Vhcl Wheel RR Trq_WhlBearing"
  Demux3/13 -> Mux/13  "Vhcl Wheel RR Trq_T2W"
  Demux3/12 -> Mux/12  "Vhcl Wheel RR SideSlip"
  Demux3/11 -> Mux/11  "Vhcl Wheel RR LongSlip"
  Demux3/10 -> Mux/10  "Vhcl Wheel RR vBelt"
  Demux3/9 -> Mux/9  "Vhcl Wheel RR Fz"
  Demux3/8 -> Mux/8  "Vhcl Wheel RR Fy"
  Demux3/7 -> Mux/7  "Vhcl Wheel RR Fx"
  Demux3/6 -> Mux/6  "Vhcl Wheel RR r_zxy z"
  Demux3/5 -> Mux/5  "Vhcl Wheel RR r_zxy y"
  Demux3/4 -> Mux/4  "Vhcl Wheel RR r_zxy x"
  Demux3/3 -> Mux/3  "Vhcl Wheel RR t z"
  Demux3/2 -> Mux/2  "Vhcl Wheel RR t y"
  Mux/1 -> Vhcl.Wheel.RR/1
  Demux3/1 -> Mux/1  "Vhcl Wheel RR t x"

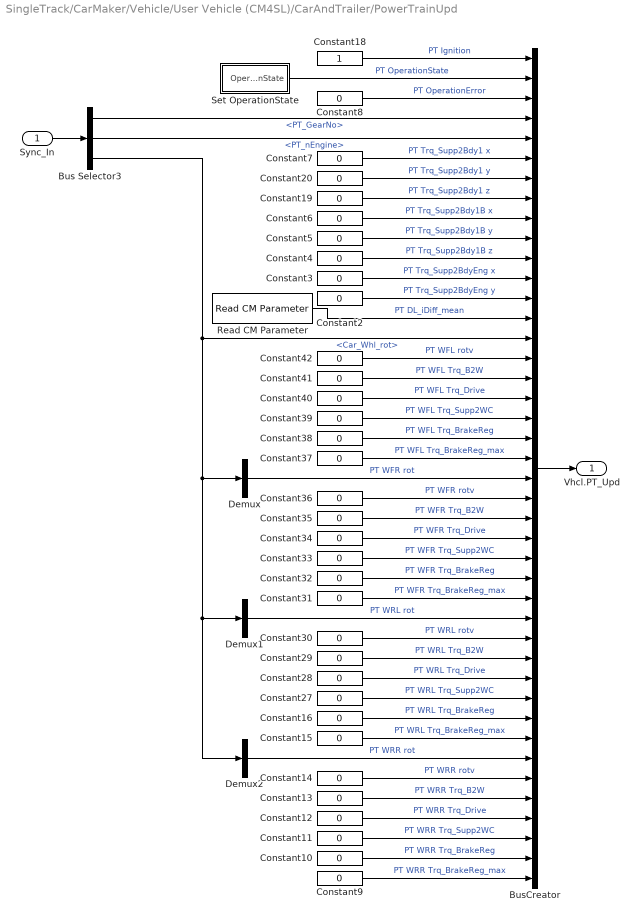
== system SingleTrack/CarMaker/Vehicle/User Vehicle (CM4SL)/CarAndTrailer/PowerTrainUpd ==
  Sync_In : Inport
  Bus Selector3 : BusSelector  OutputSignals=PT_GearNo,PT_nEngine,Car_Whl_rot
  BusCreator : BusCreator  Inputs=42
  Constant{2..16,19..20,27..42} (33 alike) : Constant  Value=0
  Constant18 : Constant
  Demux : Demux  Outputs=1
  Demux1 : Demux  Outputs=1
  Demux2 : Demux  Outputs=1
  Read CM Parameter : CarMaker4SL/Read CM Parameter  xfile=Vehicle  xkey=PowerTrain.DL.iDiff  xnout=1  xdefaults=1  xmuxed=off
  Set OperationState : Subsystem
  Vhcl.PT_Upd : Outport
  wires:
  BusCreator/1 -> Vhcl.PT_Upd/1
  Constant18/1 -> BusCreator/1  "PT Ignition"
  Set OperationState/1(OperationState) -> BusCreator/2  "PT OperationState"
  Constant8/1 -> BusCreator/3  "PT OperationError"
  Constant7/1 -> BusCreator/6  "PT Trq_Supp2Bdy1 x"
  Bus Selector3/3 -> Demux2/1, Demux1/1, Demux/1, BusCreator/15  "<Car_Whl_rot>"
  Bus Selector3/1 -> BusCreator/4  "<PT_GearNo>"
  Bus Selector3/2 -> BusCreator/5  "<PT_nEngine>"
  Sync_In/1 -> Bus Selector3/1
  Constant20/1 -> BusCreator/7  "PT Trq_Supp2Bdy1 y"
  Constant19/1 -> BusCreator/8  "PT Trq_Supp2Bdy1 z"
  Constant6/1 -> BusCreator/9  "PT Trq_Supp2Bdy1B x"
  Constant5/1 -> BusCreator/10  "PT Trq_Supp2Bdy1B y"
  Constant4/1 -> BusCreator/11  "PT Trq_Supp2Bdy1B z"
  Constant3/1 -> BusCreator/12  "PT Trq_Supp2BdyEng x"
  Constant2/1 -> BusCreator/13  "PT Trq_Supp2BdyEng y"
  Read CM Parameter/1 -> BusCreator/14  "PT DL_iDiff_mean"
  Constant42/1 -> BusCreator/16  "PT WFL rotv"
  Constant41/1 -> BusCreator/17  "PT WFL Trq_B2W"
  Constant40/1 -> BusCreator/18  "PT WFL Trq_Drive"
  Constant39/1 -> BusCreator/19  "PT WFL Trq_Supp2WC"
  Constant38/1 -> BusCreator/20  "PT WFL Trq_BrakeReg"
  Constant37/1 -> BusCreator/21  "PT WFL Trq_BrakeReg_max"
  Demux/1 -> BusCreator/22  "PT WFR rot"
  Constant36/1 -> BusCreator/23  "PT WFR rotv"
  Constant35/1 -> BusCreator/24  "PT WFR Trq_B2W"
  Constant34/1 -> BusCreator/25  "PT WFR Trq_Drive"
  Constant33/1 -> BusCreator/26  "PT WFR Trq_Supp2WC"
  Constant32/1 -> BusCreator/27  "PT WFR Trq_BrakeReg"
  Constant31/1 -> BusCreator/28  "PT WFR Trq_BrakeReg_max"
  Demux1/1 -> BusCreator/29  "PT WRL rot"
  Constant30/1 -> BusCreator/30  "PT WRL rotv"
  Constant29/1 -> BusCreator/31  "PT WRL Trq_B2W"
  Constant28/1 -> BusCreator/32  "PT WRL Trq_Drive"
  Constant27/1 -> BusCreator/33  "PT WRL Trq_Supp2WC"
  Constant16/1 -> BusCreator/34  "PT WRL Trq_BrakeReg"
  Constant15/1 -> BusCreator/35  "PT WRL Trq_BrakeReg_max"
  Demux2/1 -> BusCreator/36  "PT WRR rot"
  Constant14/1 -> BusCreator/37  "PT WRR rotv"
  Constant13/1 -> BusCreator/38  "PT WRR Trq_B2W"
  Constant12/1 -> BusCreator/39  "PT WRR Trq_Drive"
  Constant11/1 -> BusCreator/40  "PT WRR Trq_Supp2WC"
  Constant10/1 -> BusCreator/41  "PT WRR Trq_BrakeReg"
  Constant9/1 -> BusCreator/42  "PT WRR Trq_BrakeReg_max"

== system SingleTrack/CarMaker/Vehicle/User Vehicle (CM4SL)/CarAndTrailer/Query Road ==
  In1 : Inport
  Bus Selector1 : BusSelector  OutputSignals=Car_Dist,Car_x,Car_y
  Bus Selector2 : BusSelector  OutputSignals=z,slope,grade,s
  Constant1 : Constant  Value=0
  Constant2 : Constant  Value=0
  IPGRoad5 : Subsystem  mask(Query IPGRoad){xname=IPGRoad, xevalmode=RouteEval XY_S, xconsiderbumps=on, xusepath=off, xwithcurve=off, xabort=on}
      mask prompts: xname "Name"; xevalmode "Mode"; xconsiderbumps "Consider bumps"; xusepath "Use path"; xwithcurve "Output curvature"; xabort "Abort when off road"
      mask help:
      | Query IPGRoad about a given location.
      | The block should be given a unique name. In case of an error this name is logged together with the error message, making it easier to identify the location of the problem.
      mask TypeOptions xevalmode: GeoEval | RouteEval ST | RouteEval XY_S | RouteEval XY_SZ
      mask Display:
      | fprintf('<< %s >>\n%s', xname, xevalmode)
      | port_label('input', 1, 'st')
      | port_label('input', 2, 'xyz')
      | port_label('output', 1, 'Geo')
      | port_label('output', 2, 'Route')
  Mux : Mux  Inputs=3
  Mux1 : Mux  Inputs=2
  Read CM Parameter : S-Function  FunctionName=read_infoparam  Parameters=xfile,xkey,xnout,xdefaults,[],xmuxed  SFunctionDeploymentMode=off  EnableBusSupport=off  mask(Read CarMaker Infofile Parameter){xfile=Vehicle, xkey=Wheel.fl.pos, xnout=1, xdefaults=0, xmuxed=on}
      mask prompts: xfile "Parameter location"; xkey "Parameter name"; xnout "Number of outputs"; xdefaults "Default value (scalar, vector [...], or empty matrix [ ])"; xmuxed "Muxed output"
      mask help: Read the first n elements of a CarMaker infofile parameter used in the current testrun. A default value may be provided in case the parameter does not exist or does not contain at least the specified number of elements. An empty matrix [ ] specified as the default value means the parameter must exist and contain the necessary number of element, otherwise an error is generated.
      mask TypeOptions xfile: SimParameters | ECUParameters | Testrun | Vehicle | VehicleExtraData | Aero | Brake | BrakeSystem | BrakeControl | Steering | SuspF | SuspR | SuspR2 | SuspF2 | SuspExtFrcs | TireFL | TireFR | TireRL | TireRR | TireRL2 | TireRR2 | TireFL2 | TireFR2 | PTControl | PTControlOSM | PowerTrain | PowerTrainXWD | PTEngineCU | PTEngine | PTMotorCU | PTMotorISG | PTMotor | PTMotor1 | PTMotor2 | PTMotor3 | PTMotor4 | PTMotor5 | PTMotor6 | PTMotor7 | PTTransmCU | PTClutch | PTGearBox | PTGearBoxM | PTGearBoxM1 | PTGearBoxM2 | PTGearBoxM3 | PTGearBoxM4 | PTGearBoxM5 | PTGearBoxM6 | PTGearBoxM7 | PTDriveLine | PTDriveLineXWD | PTBatteryCU | PTPowerSupply | PTGenCoupling_Front | PTGenCoupling_Rear | PTGenCoupling_Center | PTGenCoupling_Rear2 | PTGenCoupling_Front2 | PTGenCoupling_HangOn | PTGenCoupling_CenterFront | PTGenCoupling_CenterRear | UserDriver | VehicleControl | VhclOperator | Trailer | TrAero | TrBrake | TrBrakeSystem | TrBrakeControl | TrSuspF | TrSuspR | TrSuspM | TrSuspExtFrcs | TrTireFL | TrTireFR | TrTireRL | TrTireRR | TrTireML | TrTireMR | Trailer2 | Tr2Aero | Tr2Brake | Tr2BrakeSystem | Tr2BrakeControl | Tr2SuspF | Tr2SuspR | Tr2SuspM | Tr2SuspExtFrcs | Tr2TireFL | Tr2TireFR | Tr2TireRL | Tr2TireRR | Tr2TireML | Tr2TireMR
      mask Display: disp(sprintf('%s\n(%s)', xkey, xfile));
  Sum2 : Sum  SaturateOnIntegerOverflow=on  InputSameDT=on  OutDataTypeStr=Inherit: Same as first input
  Terminator : Terminator
  neg : Gain  Gain=-1  SaturateOnIntegerOverflow=on  OutDataTypeStr=Inherit: Same as input  ParamDataTypeStr=Inherit: Same as input
  Fr1_z : Outport
  Fr1_rx : Outport  Port=2
  Fr1_ry : Outport  Port=3
  sRoad : Outport  Port=4
  wires:
  IPGRoad5/1(rOutGeo) -> Terminator/1
  Mux1/1 -> IPGRoad5/1(rIn.st)
  Read CM Parameter/1 -> Sum2/2
  Sum2/1 -> sRoad/1
  Bus Selector2/4 -> Sum2/1  "<s>"
  neg/1 -> Fr1_ry/1
  Bus Selector2/3 -> neg/1  "<grade>"
  Constant1/1 -> Mux1/2
  IPGRoad5/2(rOutRoute) -> Bus Selector2/1
  Bus Selector1/2 -> Mux/1  "<Car_x>"
  Bus Selector1/3 -> Mux/2  "<Car_y>"
  Mux/1 -> IPGRoad5/2(rIn.xyz)
  Bus Selector1/1 -> Mux1/1  "<Car_Dist>"
  In1/1 -> Bus Selector1/1
  Bus Selector2/1 -> Fr1_z/1  "<z>"
  Bus Selector2/2 -> Fr1_rx/1  "<slope>"
  Constant2/1 -> Mux/3

== system SingleTrack/CarMaker/Vehicle/User Vehicle (CM4SL)/CarAndTrailer/SimStates ==
  note: Detect CarMaker states and transistions relevant for initialization at the start of a new testrun.
  Logical Operator : Logic  AllPortsSameDT=off  OutDataTypeStr=boolean
  Logical Operator1 : Logic  Operator=OR  AllPortsSameDT=off  OutDataTypeStr=boolean
  Memory : Memory
  Read CM Dict : S-Function  FunctionName=read_dict  Parameters=xname, xsync  SFunctionDeploymentMode=off  EnableBusSupport=off  mask(Read CarMaker Dictionary Variable(s)){xname=SC.State, xsync=off}
      mask prompts: xname "Variable Name"; xsync "Show Sync Port"
      mask help: Copy the value(s) of the specified variable(s) of the CarMaker data dictionary to the block's output port(s). Separate the names of the variables with commas.
      mask Display: disp(xname)
  Read CM Dict1 : S-Function  FunctionName=read_dict  Parameters=xname, xsync  SFunctionDeploymentMode=off  EnableBusSupport=off  mask(Read CarMaker Dictionary Variable(s)){xname=Time, xsync=off}
      mask prompts: xname "Variable Name"; xsync "Show Sync Port"
      mask help: Copy the value(s) of the specified variable(s) of the CarMaker data dictionary to the block's output port(s). Separate the names of the variables with commas.
      mask Display: disp(xname)
  Relational Operator : RelationalOperator  Operator=<=  OutDataTypeStr=boolean
  Relational Operator1 : RelationalOperator  Operator===  OutDataTypeStr=boolean
  Relational Operator2 : RelationalOperator  Operator===  OutDataTypeStr=boolean
  SCState_Simulate : Constant  Value=8
  Zero : Constant  Value=0
  detect increase : RelationalOperator  Operator=>  OutDataTypeStr=boolean
  tag scope: TRSim=global, TRStart=global
  wires:
  Memory/1 -> detect increase/2
  detect increase/1 -> Logical Operator/1
  Logical Operator1/1 -> [TRStart]
  Logical Operator/1 -> Logical Operator1/2
  Relational Operator2/1 -> Logical Operator1/1
  Zero/1 -> Relational Operator2/2
  Read CM Dict1/1 -> Relational Operator2/1
  Relational Operator1/1 -> [TRSim]
  Relational Operator/1 -> Logical Operator/2
  SCState_Simulate/1 -> Relational Operator1/1, Relational Operator/2
  Read CM Dict/1 -> detect increase/1, Memory/1, Relational Operator1/2, Relational Operator/1

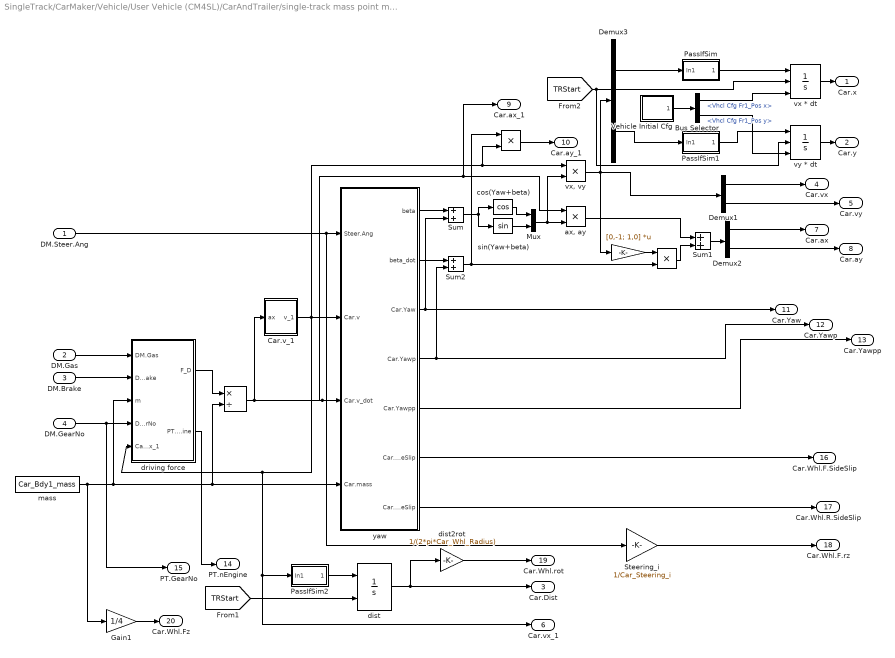
== system SingleTrack/CarMaker/Vehicle/User Vehicle (CM4SL)/CarAndTrailer/single-track mass point model ==
  DM.Steer.Ang : Inport
  DM.Gas : Inport  Port=2
  DM.Brake : Inport  Port=3
  DM.GearNo : Inport  Port=4
  " " : Gain  Gain=[0,-1; 1,0]  Multiplication=Matrix(K*u)  SaturateOnIntegerOverflow=on  OutDataTypeStr=Inherit: Same as input  ParamDataTypeStr=Inherit: Same as input
  "   " : Product  SaturateOnIntegerOverflow=on  InputSameDT=on  OutDataTypeStr=Inherit: Same as first input
  "     " : Product  SaturateOnIntegerOverflow=on  InputSameDT=on  OutDataTypeStr=Inherit: Same as first input
  "      " : Product  Inputs=*/  SaturateOnIntegerOverflow=on  InputSameDT=on  OutDataTypeStr=Inherit: Same as first input
  Bus Selector : BusSelector  OutputSignals=Vhcl Cfg Fr1_Pos x,Vhcl Cfg Fr1_Pos y
  Car.v_1 : Subsystem
  Demux1 : Demux  Outputs=2
  Demux2 : Demux  Outputs=2
  Demux3 : Demux  Outputs=2
  Gain1 : Gain  Gain=1/4
  Mux : Mux  Inputs=2
  PassIfSim : Subsystem
  PassIfSim1 : Subsystem
  PassIfSim2 : Subsystem
  "Steering_i " : Gain  Gain=1/Car_Steering_i  SaturateOnIntegerOverflow=on  OutDataTypeStr=Inherit: Same as input  ParamDataTypeStr=Inherit: Same as input
  Sum : Sum  SaturateOnIntegerOverflow=on  InputSameDT=on  OutDataTypeStr=Inherit: Same as first input
  Sum1 : Sum  SaturateOnIntegerOverflow=on  InputSameDT=on  OutDataTypeStr=Inherit: Same as first input
  Sum2 : Sum  SaturateOnIntegerOverflow=on  InputSameDT=on  OutDataTypeStr=Inherit: Same as first input
  Vehicle Initial Cfg : Subsystem  mask(Vehicle Initial Configuration Values){}
      mask help: Provides some initial vehicle configuration values.
  "ax, ay" : Product  SaturateOnIntegerOverflow=on  InputSameDT=on  OutDataTypeStr=Inherit: Same as first input
  cos(Yaw+beta) : Trigonometry  Operator=cos
  dist : Integrator  ExternalReset=level
  dist2rot : Gain  Gain=1/(2*pi*Car_Whl_Radius)  SaturateOnIntegerOverflow=on  OutDataTypeStr=Inherit: Same as input  ParamDataTypeStr=Inherit: Same as input
  driving force : Subsystem
  mass : Constant  Value=Car_Bdy1_mass
  sin(Yaw+beta) : Trigonometry
  vx * dt : Integrator  ExternalReset=level  InitialConditionSource=external  InitialCondition=[0,0]
  "vx, vy" : Product  SaturateOnIntegerOverflow=on  InputSameDT=on  OutDataTypeStr=Inherit: Same as first input
  vy * dt : Integrator  ExternalReset=level  InitialConditionSource=external  InitialCondition=[0,0]
  yaw : Subsystem
  Car.x : Outport
  Car.y : Outport  Port=2
  Car.Dist : Outport  Port=3
  Car.vx : Outport  Port=4
  Car.vy : Outport  Port=5
  Car.vx_1 : Outport  Port=6
  Car.ax : Outport  Port=7
  Car.ay : Outport  Port=8
  Car.ax_1 : Outport  Port=9
  Car.ay_1 : Outport  Port=10
  "Car.Yaw " : Outport  Port=11
  Car.Yawp : Outport  Port=12
  Car.Yawpp : Outport  Port=13
  PT.nEngine : Outport  Port=14
  PT.GearNo : Outport  Port=15
  Car.Whl.F.SideSlip : Outport  Port=16
  Car.Whl.R.SideSlip : Outport  Port=17
  Car.Whl.F.rz : Outport  Port=18
  Car.Whl.rot : Outport  Port=19
  Car.Whl.Fz : Outport  Port=20
  wires:
  Gain1/1 -> Car.Whl.Fz/1
  Bus Selector/1 -> vx * dt/3  "<Vhcl Cfg Fr1_Pos x>"
  Bus Selector/2 -> vy * dt/3  "<Vhcl Cfg Fr1_Pos y>"
  Vehicle Initial Cfg/1(Vhcl.Cfg) -> Bus Selector/1
  vx * dt/1 -> Car.x/1
  vy * dt/1 -> Car.y/1
  [TRStart] -> vy * dt/2, vx * dt/2
  yaw/1(beta) -> Sum/1
  yaw/3(Car.Yaw) -> Sum/2, "Car.Yaw "/1
  cos(Yaw+beta)/1 -> Mux/1
  sin(Yaw+beta)/1 -> Mux/2
  Sum/1 -> cos(Yaw+beta)/1, sin(Yaw+beta)/1
  yaw/5(Car.Yawpp) -> Car.Yawpp/1
  yaw/4(Car.Yawp) -> Car.Yawp/1, Sum2/2
  Mux/1 -> "ax, ay"/2, "vx, vy"/2
  "vx, vy"/1 -> Demux3/1, Demux1/1, " "/1
  Car.v_1/1(v_1) -> yaw/2(Car.v), "vx, vy"/1, "     "/2, driving force/5(Car.vx_1), Car.vx_1/1, PassIfSim2/1(In1)
  Sum1/1 -> Demux2/1
  "   "/1 -> Sum1/2
  "ax, ay"/1 -> Sum1/1
  yaw/2(beta_dot) -> Sum2/1
  Sum2/1 -> "   "/2, "     "/1
  " "/1 -> "   "/1
  "     "/1 -> Car.ay_1/1
  DM.Steer.Ang/1 -> yaw/1(Steer.Ang), "Steering_i "/1
  yaw/6(Car.Whl.F.SideSlip) -> Car.Whl.F.SideSlip/1
  yaw/7(Car.Whl.SideSlip) -> Car.Whl.R.SideSlip/1
  "      "/1 -> Car.v_1/1(ax), yaw/3(Car.v_dot), Car.ax_1/1, "ax, ay"/1
  driving force/1(F_D) -> "      "/1
  DM.Brake/1 -> driving force/2(DM.Brake)
  DM.Gas/1 -> driving force/1(DM.Gas)
  Demux1/2 -> Car.vy/1
  Demux2/1 -> Car.ax/1
  Demux2/2 -> Car.ay/1
  dist/1 -> Car.Dist/1, dist2rot/1
  Demux1/1 -> Car.vx/1
  DM.GearNo/1 -> driving force/4(DM.GearNo), PT.GearNo/1
  mass/1 -> Gain1/1, driving force/3(m), yaw/4(Car.mass), "      "/2
  driving force/2(PT.nEngine) -> PT.nEngine/1
  "Steering_i "/1 -> Car.Whl.F.rz/1
  dist2rot/1 -> Car.Whl.rot/1
  Demux3/1 -> PassIfSim/1(In1)
  PassIfSim/1(Out1) -> vx * dt/1
  Demux3/2 -> PassIfSim1/1(In1)
  PassIfSim1/1(Out1) -> vy * dt/1
  PassIfSim2/1(Out1) -> dist/1
  [TRStart] -> dist/2

== system SingleTrack/CarMaker/Vehicle/User Vehicle (ModelMgr)/Brake/CreateBus Vhcl.Wheel.PT ==
  In : Inport
  BusCreator1 : BusCreator  Inputs=20
  Demux1 : Demux  Outputs=20
  Out : Outport
  wires:
  Demux1/20 -> BusCreator1/20  "Vhcl Trq_DriveSrc_trg d3"
  Demux1/19 -> BusCreator1/19  "Vhcl Trq_DriveSrc_trg d2"
  Demux1/18 -> BusCreator1/18  "Vhcl Trq_DriveSrc_trg d1"
  Demux1/17 -> BusCreator1/17  "Vhcl Trq_DriveSrc_trg d0"
  Demux1/16 -> BusCreator1/16  "Vhcl Wheel RR WhlBearing"
  Demux1/15 -> BusCreator1/15  "Vhcl Wheel RR Trq_T2W"
  Demux1/14 -> BusCreator1/14  "Vhcl Wheel RR Trq_BrakeReg_trg"
  Demux1/13 -> BusCreator1/13  "Vhcl Wheel RR Trq_Brake"
  Demux1/12 -> BusCreator1/12  "Vhcl Wheel RL WhlBearing"
  Demux1/11 -> BusCreator1/11  "Vhcl Wheel RL Trq_T2W"
  Demux1/10 -> BusCreator1/10  "Vhcl Wheel RL Trq_BrakeReg_trg"
  Demux1/9 -> BusCreator1/9  "Vhcl Wheel RL Trq_Brake"
  Demux1/8 -> BusCreator1/8  "Vhcl Wheel FR WhlBearing"
  Demux1/7 -> BusCreator1/7  "Vhcl Wheel FR Trq_T2W"
  Demux1/6 -> BusCreator1/6  "Vhcl Wheel FR Trq_BrakeReg_trg"
  Demux1/5 -> BusCreator1/5  "Vhcl Wheel FR Trq_Brake"
  Demux1/4 -> BusCreator1/4  "Vhcl Wheel FL WhlBearing"
  Demux1/3 -> BusCreator1/3  "Vhcl Wheel FL Trq_T2W"
  Demux1/2 -> BusCreator1/2  "Vhcl Wheel FL Trq_BrakeReg_trg"
  Demux1/1 -> BusCreator1/1  "Vhcl Wheel FL Trq_Brake"
  BusCreator1/1 -> Out/1
  In/1 -> Demux1/1

== system SingleTrack/CarMaker/Vehicle/User Vehicle (ModelMgr)/CarAndTrailer/CarAndTrailerUpd ==
  Sync_In : Inport
  Vhcl.Steering : Inport  Port=2
  Vhcl.Motion : Inport  Port=3
  Vhcl.PoI : Inport  Port=4
  Vhcl.Wheel.FL : Inport  Port=5
  Vhcl.Wheel.FR : Inport  Port=6
  Vhcl.Wheel.RL : Inport  Port=7
  Vhcl.Wheel.RR : Inport  Port=8
  Car.Hitch.FrcTrq : Inport  Port=9
  Vhcl.Fr1A : Inport  Port=10
  CarAndTrailerUpd : S-Function  FunctionName=CM_Sfun  Parameters='CarAndTrUpd'  SFunctionDeploymentMode=off  EnableBusSupport=off
  CreateBus Brake.IF.In : Subsystem
  Sync_Out : Outport
  Brake.IF.In : Outport  Port=2
  wires:
  Vhcl.Fr1A/1 -> CarAndTrailerUpd/10  "user vehicle only"
  Vhcl.Steering/1 -> CarAndTrailerUpd/2
  Vhcl.Motion/1 -> CarAndTrailerUpd/3
  Vhcl.PoI/1 -> CarAndTrailerUpd/4
  Vhcl.Wheel.FL/1 -> CarAndTrailerUpd/5
  Vhcl.Wheel.FR/1 -> CarAndTrailerUpd/6
  Car.Hitch.FrcTrq/1 -> CarAndTrailerUpd/9
  Vhcl.Wheel.RR/1 -> CarAndTrailerUpd/8
  Vhcl.Wheel.RL/1 -> CarAndTrailerUpd/7
  CarAndTrailerUpd/2 -> CreateBus Brake.IF.In/1(In)
  CreateBus Brake.IF.In/1(Out) -> Brake.IF.In/1
  CarAndTrailerUpd/1 -> Sync_Out/1
  Sync_In/1 -> CarAndTrailerUpd/1

== system SingleTrack/CarMaker/Vehicle/IPG Vehicle/CarAndTrailer/CarAndTrailerUpd/CreateBus Brake.IF.In ==
  In : Inport
  BusCreator : BusCreator  Inputs=9
  Demux : Demux  Outputs=9
  Out : Outport
  wires:
  Demux/9 -> BusCreator/9  "Brake IF Trq_Reg RR"
  Demux/8 -> BusCreator/8  "Brake IF Trq_Reg RL"
  Demux/7 -> BusCreator/7  "Brake IF Trq_Reg FR"
  Demux/6 -> BusCreator/6  "Brake IF Trq_Reg FL"
  Demux/5 -> BusCreator/5  "Brake IF Trq_Reg_max RR"
  Demux/4 -> BusCreator/4  "Brake IF Trq_Reg_max RL"
  Demux/3 -> BusCreator/3  "Brake IF Trq_Reg_max FR"
  Demux/2 -> BusCreator/2  "Brake IF Trq_Reg_max FL"
  Demux/1 -> BusCreator/1  "Brake IF T_env"
  BusCreator/1 -> Out/1
  In/1 -> Demux/1

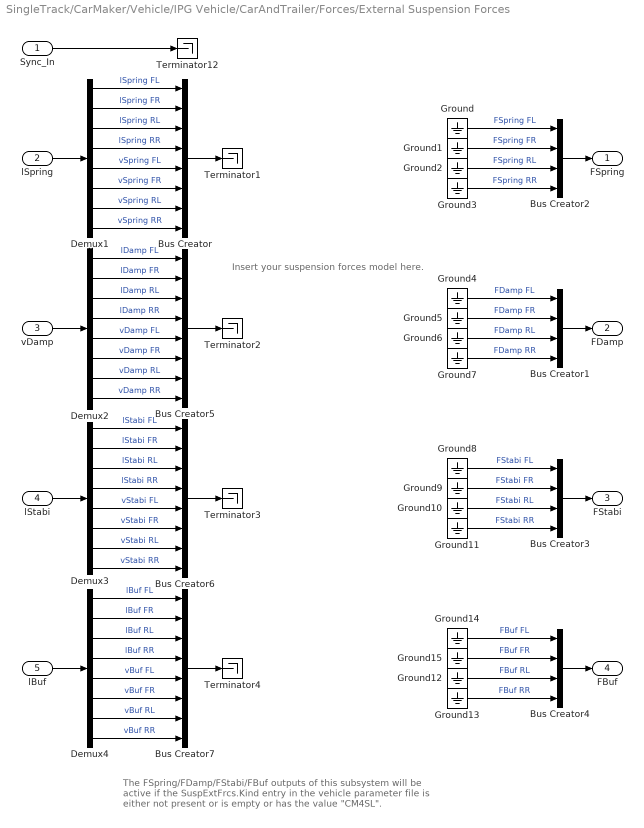
== system SingleTrack/CarMaker/Vehicle/IPG Vehicle/CarAndTrailer/Forces/External Suspension Forces ==
  note: The FSpring/FDamp/FStabi/FBuf outputs of this subsystem will be
      | active if the SuspExtFrcs.Kind entry in the vehicle parameter file
      | is either not present or is empty or has the value "CM4SL".
  note: Insert your suspension forces model here.
  Sync_In : Inport
  lSpring : Inport  Port=2
  vDamp : Inport  Port=3
  lStabi : Inport  Port=4
  lBuf : Inport  Port=5
  Bus Creator{,5..7} (4 alike) : BusCreator  Inputs=8
  Bus Creator{1..4} (4 alike) : BusCreator  Inputs=4
  Demux{1..4} (4 alike) : Demux  Outputs=8
  Ground{,1..15} (16 alike) : Ground
  Terminator{1..4,12} (5 alike) : Terminator
  FSpring : Outport
  FDamp : Outport  Port=2
  FStabi : Outport  Port=3
  FBuf : Outport  Port=4
  wires:
  Bus Creator7/1 -> Terminator4/1
  Bus Creator6/1 -> Terminator3/1
  Bus Creator5/1 -> Terminator2/1
  Bus Creator/1 -> Terminator1/1
  Demux4/8 -> Bus Creator7/8  "vBuf RR"
  Demux4/7 -> Bus Creator7/7  "vBuf RL"
  Demux4/6 -> Bus Creator7/6  "vBuf FR"
  Demux4/5 -> Bus Creator7/5  "vBuf FL"
  Demux3/8 -> Bus Creator6/8  "vStabi RR"
  Demux3/7 -> Bus Creator6/7  "vStabi RL"
  Demux3/6 -> Bus Creator6/6  "vStabi FR"
  Demux3/5 -> Bus Creator6/5  "vStabi FL"
  Demux2/8 -> Bus Creator5/8  "vDamp RR"
  Demux2/7 -> Bus Creator5/7  "vDamp RL"
  Demux2/6 -> Bus Creator5/6  "vDamp FR"
  Demux2/5 -> Bus Creator5/5  "vDamp FL"
  Demux1/8 -> Bus Creator/8  "vSpring RR"
  Demux1/7 -> Bus Creator/7  "vSpring RL"
  Demux1/6 -> Bus Creator/6  "vSpring FR"
  Demux1/5 -> Bus Creator/5  "vSpring FL"
  Demux2/4 -> Bus Creator5/4  "lDamp RR"
  Demux2/3 -> Bus Creator5/3  "lDamp RL"
  Demux2/2 -> Bus Creator5/2  "lDamp FR"
  Demux2/1 -> Bus Creator5/1  "lDamp FL"
  Demux1/4 -> Bus Creator/4  "lSpring RR"
  Demux1/3 -> Bus Creator/3  "lSpring RL"
  Demux1/2 -> Bus Creator/2  "lSpring FR"
  Demux1/1 -> Bus Creator/1  "lSpring FL"
  Demux3/4 -> Bus Creator6/4  "lStabi RR"
  Demux3/3 -> Bus Creator6/3  "lStabi RL"
  Demux3/2 -> Bus Creator6/2  "lStabi FR"
  Demux3/1 -> Bus Creator6/1  "lStabi FL"
  lStabi/1 -> Demux3/1
  vDamp/1 -> Demux2/1
  lSpring/1 -> Demux1/1
  Demux4/4 -> Bus Creator7/4  "lBuf RR"
  Demux4/3 -> Bus Creator7/3  "lBuf RL"
  Demux4/2 -> Bus Creator7/2  "lBuf FR"
  Demux4/1 -> Bus Creator7/1  "lBuf FL"
  lBuf/1 -> Demux4/1
  Ground14/1 -> Bus Creator4/1  "FBuf FL"
  Ground15/1 -> Bus Creator4/2  "FBuf FR"
  Ground12/1 -> Bus Creator4/3  "FBuf RL"
  Ground13/1 -> Bus Creator4/4  "FBuf RR"
  Bus Creator4/1 -> FBuf/1
  Sync_In/1 -> Terminator12/1
  Bus Creator2/1 -> FSpring/1
  Ground/1 -> Bus Creator2/1  "FSpring FL"
  Ground1/1 -> Bus Creator2/2  "FSpring FR"
  Ground2/1 -> Bus Creator2/3  "FSpring RL"
  Ground3/1 -> Bus Creator2/4  "FSpring RR"
  Ground4/1 -> Bus Creator1/1  "FDamp FL"
  Ground5/1 -> Bus Creator1/2  "FDamp FR"
  Ground6/1 -> Bus Creator1/3  "FDamp RL"
  Ground7/1 -> Bus Creator1/4  "FDamp RR"
  Bus Creator1/1 -> FDamp/1
  Ground8/1 -> Bus Creator3/1  "FStabi FL"
  Ground9/1 -> Bus Creator3/2  "FStabi FR"
  Ground10/1 -> Bus Creator3/3  "FStabi RL"
  Ground11/1 -> Bus Creator3/4  "FStabi RR"
  Bus Creator3/1 -> FStabi/1
